simulink subsystem "Check_Quat"  (R2023a)
settings: Solver=VariableStepAuto  StartTime=0.0  StopTime=10.0  RelTol=1e-3
libraries: sharedutil x1
settings Model: Creator=thesa  LastModifiedBy=thesa

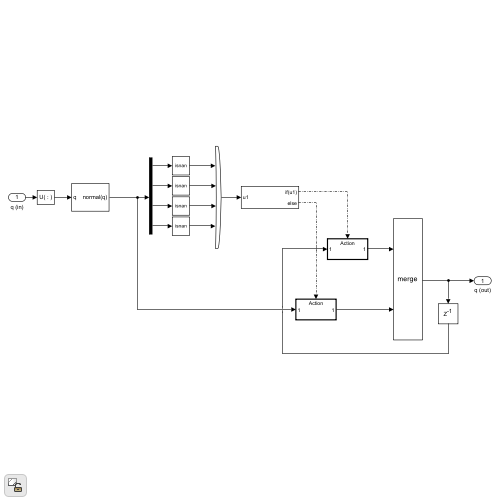
[thumbnail: Simulink's stored preview of the top-level diagram]
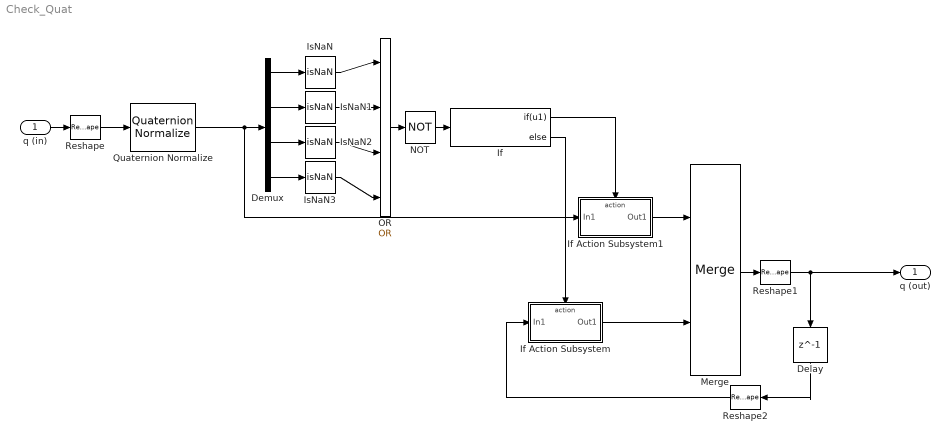
== system Check_Quat ==
  q (in) : Inport
  Delay : Delay  DelayLength=1  InitialCondition=[1,0,0,0]
  Demux : Demux
  If : If  IfExpression=u1
  If Action Subsystem : Subsystem  TreatAsAtomicUnit=on
  If Action Subsystem1 : Subsystem  TreatAsAtomicUnit=on
  IsNaN{,1..3} (4 alike) : RelationalOperator  Operator=isNaN  OutDataTypeStr=boolean  RndMeth=Simplest  InputSameDT=off
  Merge : Merge
  NOT : Logic  Operator=NOT  IconShape=distinctive  AllPortsSameDT=off  OutDataTypeStr=boolean
  OR : Logic  Operator=OR  Inputs=4  IconShape=distinctive  AllPortsSameDT=off  OutDataTypeStr=boolean
  Quaternion Normalize : sharedutil/Quaternion Normalize  aMode=aMode
  Reshape : Reshape
  Reshape1 : Reshape  OutputDimensionality=Row vector (2-D)
  Reshape2 : Reshape
  q (out) : Outport
  wires:
  q (in)/1 -> Reshape/1
  Demux/2 -> IsNaN1/1
  IsNaN1/1 -> OR/2
  Demux/1 -> IsNaN/1
  Reshape/1 -> Quaternion Normalize/1
  IsNaN3/1 -> OR/4
  Merge/1 -> Reshape1/1
  Demux/3 -> IsNaN2/1
  Quaternion Normalize/1 -> If Action Subsystem1/1(In1), Demux/1
  IsNaN2/1 -> OR/3
  OR/1 -> NOT/1
  IsNaN/1 -> OR/1
  Demux/4 -> IsNaN3/1
  Delay/1 -> Reshape2/1
  Reshape1/1 -> Delay/1, q (out)/1
  NOT/1 -> If/1
  If/1 -> If Action Subsystem1/Action
  If Action Subsystem/1(Out1) -> Merge/2
  If Action Subsystem1/1(Out1) -> Merge/1
  If/2 -> If Action Subsystem/Action
  Reshape2/1 -> If Action Subsystem/1(In1)

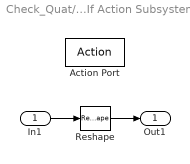
== system Check_Quat/If Action Subsystem ==
  In1 : Inport
  Action Port : ActionPort
  Reshape : Reshape
  Out1 : Outport
  wires:
  In1/1 -> Reshape/1
  Reshape/1 -> Out1/1

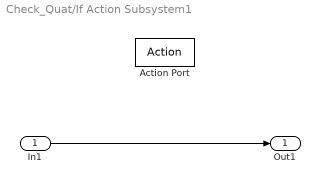
== system Check_Quat/If Action Subsystem1 ==
  In1 : Inport
  Action Port : ActionPort
  Out1 : Outport
  wires:
  In1/1 -> Out1/1
